simulink model "DC_Motor_Modeling"  (R2025a)
settings: Solver=VariableStepAuto  StartTime=0.0  StopTime=3  RelTol=1e-3
values from neighbouring files (symbols this model uses):
  B_m = (kfi^2*I_anl)/(V_an-R_a*I_anl)    (= 1.14618667775e-06)    [DC_Motor_Modeling.m]
  den_sim = [(J_m*L_a) (J_m*R_a+B_m*L_a) (B_m*R_a+kfi^2)]    [DC_Motor_Modeling.m]
  den_sim_current = [(J_m*L_a) (J_m*R_a+B_m*L_a) (B_m*R_a+kfi^2)]    [DC_Motor_Modeling.m]
  J_m = 8.85*10^-7    (= 8.85e-07)    [DC_Motor_Modeling.m]
  kfi = 0.0453    [DC_Motor_Modeling.m]
  L_a = 0.746*10^-3    (= 0.000746)    [DC_Motor_Modeling.m]
  num_sim = [kfi]    [DC_Motor_Modeling.m]
  num_sim_current = [J_m B_m]    [DC_Motor_Modeling.m]
  R_a = 7.39    [DC_Motor_Modeling.m]
  T_n = 28.9*10^-3    (= 0.0289)    [DC_Motor_Modeling.m]
  T_s = 294*10^-3    (= 0.294)    [DC_Motor_Modeling.m]
  V_an = 48    [DC_Motor_Modeling.m]
libraries: spsDCMachineLib x1, spsDCVoltageSourceLib x1, sps_lib x1
settings Model: Creator=DE MK - EN  LastModifiedBy=Chrisson

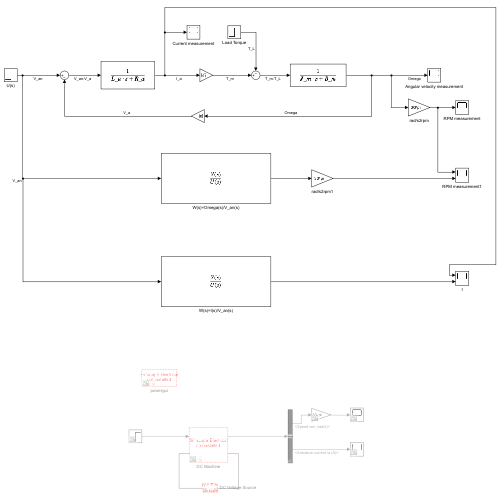
[thumbnail: Simulink's stored preview of the top-level diagram]
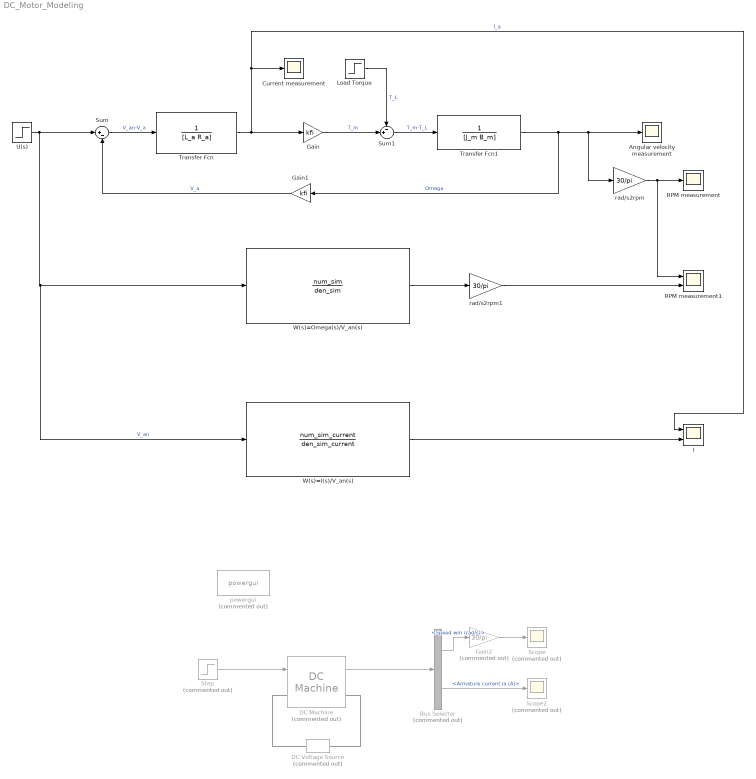
== system DC_Motor_Modeling ==
  Angular velocity measurement : Scope
      settings: ActiveDisplayYMinimum=-131.91004  ActiveDisplayYMaximum=1187.19039
  Bus Selector : BusSelector  Commented=on  OutputSignals=Speed wm (rad/s),Armature current ia (A)
  Current measurement : Scope
      settings: Title=Motor Current  ActiveDisplayYMinimum=-0.81216  ActiveDisplayYMaximum=7.30948  YLabel=Current(A)
  DC Machine : spsDCMachineLib/DC Machine  Commented=on  PresetModel=No  MechanicalLoad=Torque TL  FieldType=Permanent magnet  ShowDetailedParameters=on  MeasurementBus=off  RLa=[R_a L_a]  RLf=[180 71.47]  Laf=0.6458  MachineConstant=Torque constant (N.m/A)  Ke=1.8  Kt=kfi  J=J_m  Bm=B_m  Tf=0  w0=0  Ifinit=1  TsPowergui=0  TsBlock=-1
  DC Voltage Source : spsDCVoltageSourceLib/DC Voltage Source  Commented=on  Amplitude=100  Measurements=None
  Gain : Gain  Gain=kfi
  Gain1 : Gain  Gain=kfi
  Gain2 : Gain  Commented=on  Gain=30/pi
  I : Scope  NumInputPorts=2
      settings: Title=Current of the motor  ActiveDisplayYMinimum=-0.81216  ActiveDisplayYMaximum=7.30948  YLabel=Current (A)  DataLoggingVariableName=ScopeData2
  Load Torque : Step  Time=2  After=T_s  SampleTime=0
  RPM measurement : Scope
      settings: Title=RPM of DC motor  ActiveDisplayYMinimum=-1259.64812  ActiveDisplayYMaximum=11336.83312  YLabel=Speed (rpm)  DataLoggingVariableName=ScopeData2
  RPM measurement1 : Scope  NumInputPorts=2
      settings: Title=RPM of DC motor  ActiveDisplayYMinimum=-1259.6479225197095  ActiveDisplayYMaximum=11336.831302677387  YLabel=Speed (rpm)
  Scope : Scope  Commented=on
      settings: Title=RPM of DC Motor  ActiveDisplayYMinimum=-2624.27411  ActiveDisplayYMaximum=23618.46702  YLabel=Speed(Rpm)
  Scope2 : Scope  Commented=on
      settings: Title=Current of DC Motor  ActiveDisplayYMinimum=-1.64482  ActiveDisplayYMaximum=15.21809  YLabel=Current(A)  DataLoggingVariableName=ScopeData3
  Step : Step  Commented=on  After=T_n  SampleTime=0
  Sum : Sum  Inputs=|+-
  Sum1 : Sum  Inputs=-+|
  Transfer Fcn : TransferFcn  Denominator=[L_a R_a]
  Transfer Fcn1 : TransferFcn  Denominator=[J_m B_m]
  U(s) : Step  After=V_an  SampleTime=0
  W(s)=I(s)/V_an(s) : TransferFcn  Numerator=num_sim_current  Denominator=den_sim_current
  W(s)=Omega(s)/V_an(s) : TransferFcn  Numerator=num_sim  Denominator=den_sim
  powergui : sps_lib/powergui  Priority=1  Commented=on  SimulationMode=Continuous  SampleTime=50e-6  frequency=60  Iterations=50  frequencyindice=0  Pbase=100e6  ErrMax=1e-4  UnitsV=kV  UnitsW=MW  buscounter=0  FunctionMessages=off  echomessages=off  EnableUseOfTLC=off  CurrentSourceSwitches=off  DisableSnubberDevices=off  DisableRonSwitches=off  DisableVfSwitches=off  DisplayEquations=off  AutomaticDiscreteSolvers=off  SolverType=Tustin/Backward Euler (TBE)  Interpol=off  ExternalGateDelay=off  methode=off  Ts=100  x0status=blocks  SPID=on  SwTol=0  HookPort=off  NonlinearTolerance=1e-4  nMaxIteration=100  ContinueOnMaxIteration=off  RestoreLinks=warning  ResistiveCurrentMeasurement=off  Frange=[0:2:500]  Ylog=off  Xlog=on  ShowGrid=off  save=off  variable=ZData  structure=0  ZoomFFT=off  StartTime=0.0  cycles=1  DisplayStyle=1  fundamental=60  FreqAxis=off  MaxFrequency=1000  frequencyindicesteady=1  RmsSteady=1  display=off
  rad/s2rpm : Gain  Gain=30/pi
  rad/s2rpm1 : Gain  Gain=30/pi
  wires:
  Sum/1 -> Transfer Fcn/1  "V_an-V_a"
  Transfer Fcn/1 -> Current measurement/1, I/1, Gain/1  "I_a"
  Transfer Fcn1/1 -> rad/s2rpm/1, Angular velocity measurement/1, Gain1/1  "Omega"
  Gain1/1 -> Sum/2  "V_a"
  Load Torque/1 -> Sum1/1  "T_L"
  Sum1/1 -> Transfer Fcn1/1  "T_m-T_L"
  Gain/1 -> Sum1/2  "T_m"
  rad/s2rpm/1 -> RPM measurement1/1, RPM measurement/1
  rad/s2rpm1/1 -> RPM measurement1/2
  W(s)=Omega(s)/V_an(s)/1 -> rad/s2rpm1/1
  U(s)/1 -> W(s)=I(s)/V_an(s)/1, W(s)=Omega(s)/V_an(s)/1, Sum/1  "V_an"
  W(s)=I(s)/V_an(s)/1 -> I/2
  Step/1 -> DC Machine/1
  DC Machine/1 -> Bus Selector/1
  Bus Selector/1 -> Gain2/1  "<Speed wm (rad/s)>"
  Bus Selector/2 -> Scope2/1  "<Armature current ia (A)>"
  Gain2/1 -> Scope/1
  connections:
  DC Machine/LConn1 -- DC Voltage Source/RConn1
  DC Machine/RConn1 -- DC Voltage Source/LConn1
